simulink model "irep_force_control_m15"  (R2015a)
settings: Solver=ode3  StartTime=0.0  StopTime=inf  FixedStep=dt  RelTol=1e-3
InitFcn:
  | IREP_DEPENDENCY
  | init_omni
  | init_filters
  | init_invivo
  | init_telemanipulation
  | init_parker_xyz
  | init_magnetic_tracker
  | init_loadcell
  | init_scopes
  | init_homing
  | init_force_control
  | init_xpc_invivo_simu
undefined symbols (not defined in the file): ang_vel_scale, B_simu, beta, camera_home_voltage, counter_offset, dt, dt_trakstar, E_Y, encoder_counts, epsilon_robust_inverse, FS_LUT_TAU, FS_LUT_WE, gear_ratio, HomingFineEps, HomingRoughEps, HomingRoughVelocity, I1_primary, I1_secondary, I2_primary, I2_secondary, irep_parameters_left, irep_parameters_right, joystick_filter_coeffs, K_d, K_i, K_naive_inv, K_p, k_right, L1l, L1r, L2l, L2r, L_zeus, left_arm_home_voltage, left_x0_parallelogram, LeftArmHomingDirectionVector, LeftArmHomingIntGain, lin_vel_scale, LOADCELL_BIAS, LOADCELL_GAIN, max_conf_space_speed, N_joystick, N_pots, N_trakstar, OmegaMax, OmegaMin, orientation_epsilon, position_epsilon, pots_filter_coeffs, q_eps_backlash, quadrature_mode, r, right_arm_home_voltage, RightArmHomingDirectionVector, RightArmHomingIntGain, screw_pitch, statics_param, tau_compression_bias, tau_compression_gains, tau_neutral_deadband ... (+16)
libraries: slrtlib x39, simulink x23, xpcobsoletelib x23, xpcconteclib x23, xpcrtudplib x12, xpcmeasurementcomputinglib x6, dspswit3 x2, dspsigops x1
(part 4 of 7)

== system irep_force_control_m15/Wrench Estimation/tau sensing compensation/tau sensing compensation gain model ==
  q_bb : Inport
  tau_sensed : Inport  Port=2
  Enable : EnablePort
  friction compensation : MATLAB Function  TreatAsAtomicUnit=on
  tau_compression_bias : Constant  Value=tau_compression_bias
  tau_compression_gains : Constant  Value=tau_compression_gains
  tau_neutral_deadband : Constant  Value=tau_neutral_deadband
  tau_tension_bias : Constant  Value=tau_tension_bias
  tau_tension_gains : Constant  Value=tau_tension_gains
  tau_comp : Outport
  wires:
  tau_neutral_deadband/1 -> friction compensation/7(deadband)
  tau_compression_gains/1 -> friction compensation/4(gain_compression)
  tau_tension_gains/1 -> friction compensation/3(gain_tension)
  tau_sensed/1 -> friction compensation/2(tau_sensed)
  q_bb/1 -> friction compensation/1(q_bb)
  friction compensation/1(tau_comp) -> tau_comp/1
  tau_tension_bias/1 -> friction compensation/5(bias_tension)
  tau_compression_bias/1 -> friction compensation/6(bias_compression)

== system irep_force_control_m15/In-Vivo System/Magnetic Tracker 125 Hz/process trak1/Filter1 ==
  in : Inport
  Discrete FIR Filter : DiscreteFir  CoefSource=Input port  SampleTime=dt_trakstar  AccumDataTypeStr=Inherit: Same as product output
  Gain : Gain  Gain=1/N_trakstar  SampleTime=dt_trakstar
  trakstar_filter_coeffs : Constant  Value=trakstar_filter_coeffs  SampleTime=dt_trakstar
  out : Outport
  wires:
  Gain/1 -> out/1
  in/1 -> Discrete FIR Filter/1
  Discrete FIR Filter/1 -> Gain/1
  trakstar_filter_coeffs/1 -> Discrete FIR Filter/2

== system irep_force_control_m15/In-Vivo System/Magnetic Tracker 125 Hz/process trak2/Filter1 ==
  in : Inport
  Discrete FIR Filter : DiscreteFir  CoefSource=Input port  SampleTime=dt_trakstar  AccumDataTypeStr=Inherit: Same as product output
  Gain : Gain  Gain=1/N_trakstar  SampleTime=dt_trakstar
  trakstar_filter_coeffs : Constant  Value=trakstar_filter_coeffs  SampleTime=dt_trakstar
  out : Outport
  wires:
  trakstar_filter_coeffs/1 -> Discrete FIR Filter/2
  Discrete FIR Filter/1 -> Gain/1
  in/1 -> Discrete FIR Filter/1
  Gain/1 -> out/1

== system irep_force_control_m15/In-Vivo System/Magnetic Tracker 125 Hz/process trak3/Filter1 ==
  in : Inport
  Discrete FIR Filter : DiscreteFir  CoefSource=Input port  SampleTime=dt_trakstar  AccumDataTypeStr=Inherit: Same as product output
  Gain : Gain  Gain=1/N_trakstar  SampleTime=dt_trakstar
  trakstar_filter_coeffs : Constant  Value=trakstar_filter_coeffs  SampleTime=dt_trakstar
  out : Outport
  wires:
  Gain/1 -> out/1
  in/1 -> Discrete FIR Filter/1
  Discrete FIR Filter/1 -> Gain/1
  trakstar_filter_coeffs/1 -> Discrete FIR Filter/2

== system irep_force_control_m15/In-Vivo System/Magnetic Tracker 125 Hz/process trak4/Filter1 ==
  in : Inport
  Discrete FIR Filter : DiscreteFir  CoefSource=Input port  SampleTime=dt_trakstar  AccumDataTypeStr=Inherit: Same as product output
  Gain : Gain  Gain=1/N_trakstar  SampleTime=dt_trakstar
  trakstar_filter_coeffs : Constant  Value=trakstar_filter_coeffs  SampleTime=dt_trakstar
  out : Outport
  wires:
  trakstar_filter_coeffs/1 -> Discrete FIR Filter/2
  Discrete FIR Filter/1 -> Gain/1
  in/1 -> Discrete FIR Filter/1
  Gain/1 -> out/1

== system irep_force_control_m15/Trajectory Planner/Left Arm/High Level/Actuation Compensation ==
  q des : Inport
  conf space : Inport  Port=2
  Enable : EnablePort
  1/stiffness : Gain  Gain=K_naive_inv  Multiplication=Matrix(K*u)  SampleTime=dt
  Compute Taus : Subsystem
  Grad U1 : Subsystem
  Grad U2 : Subsystem
  Mux : Mux  Inputs=2
  Mux1 : Mux  Inputs=3
  Parallelogram Backlash Compensatior : Subsystem  TreatAsAtomicUnit=on
  comp perc : Gain  Gain=diag([0.8 0.8 0.8 0.8])  Multiplication=Matrix(K*u)  SampleTime=dt
  padding 2 for wrist and gripper : Constant  Value=zeros(2,1)  SampleTime=dt
  epsilon : Outport
  wires:
  conf space/1 -> Grad U1/1(conf space), Compute Taus/2(In2), Grad U2/1(conf space)
  q des/1 -> Grad U2/2(q), Grad U1/2(q), Parallelogram Backlash Compensatior/1(q des)
  Grad U1/1(grad_U) -> Mux/1
  Grad U2/1(grad_U) -> Mux/2
  Mux/1 -> Compute Taus/1(In1)
  Compute Taus/1(tau) -> 1/stiffness/1
  Parallelogram Backlash Compensatior/1(epsilon) -> Mux1/1
  1/stiffness/1 -> comp perc/1  "epsilon"
  padding 2 for wrist and gripper/1 -> Mux1/3
  comp perc/1 -> Mux1/2
  Mux1/1 -> epsilon/1

== system irep_force_control_m15/Trajectory Planner/Left Arm/High Level/Configuration Space ==
  Enable : EnablePort
  Enable Parallelogram : Constant  Value=0  SampleTime=dt
  Enable Stem : Constant  Value=0  SampleTime=dt
  Mux : Mux  Inputs=3
  Parallelogram : Subsystem  TreatAsAtomicUnit=on
  Stem : Subsystem  TreatAsAtomicUnit=on
  b0 : Constant  Value=0  SampleTime=dt
  "b1 dot, psi dot" : Outport  InitialOutput=zeros(8,1)
  wires:
  Enable Stem/1 -> Stem/Enable
  Enable Parallelogram/1 -> Parallelogram/Enable
  Mux/1 -> "b1 dot, psi dot"/1
  b0/1 -> Mux/1
  Parallelogram/1(b1) -> Mux/2
  Stem/1(psi dot) -> Mux/3

== system irep_force_control_m15/Trajectory Planner/Left Arm/High Level/Inverse Istantaneous Kinematics ==
  In1 : Inport
  sensors : Inport  Port=2
  Master : Inport  Port=3
  5-Bar Inverse Kinematics : MATLAB Function  TreatAsAtomicUnit=on
  Bus Creator : BusCreator  Inputs=3
  Bus Creator1 : BusCreator
  Bus Selector : BusSelector  OutputSignals=q.Parker insertion stage
  Coordination Module : Subsystem
  Demux : Demux  Outputs=[1 2 5]
  Enable Gripper : Constant  Value=0  SampleTime=dt
  Integrator 3 : DiscreteIntegrator  InitialCondition=[left_x0_parallelogram z0_parallelogram]  SampleTime=dt  LimitOutput=on  UpperSaturationLimit=[-x0_parallelogram z0_parallelogram_max]  LowerSaturationLimit=[-x0_parallelogram_max z0_parallelogram]
  Integrator 4 : DiscreteIntegrator  InitialCondition=[pi/2;0;pi/2;0;0]  SampleTime=dt  LimitOutput=on  UpperSaturationLimit=[theta_max inf theta_max inf wrist_max]  LowerSaturationLimit=[theta_min1 -inf theta_min2 -inf wrist_min]
  Jaw Open/Close Module : Subsystem  TreatAsAtomicUnit=on
  Saturation : Saturate  UpperLimit=20  LowerLimit=0
  Snake inverse kinematics : MATLAB Function  TreatAsAtomicUnit=on
  q des : Outport
  conf space : Outport  Port=2
  b0 dot left : Outport  Port=3
  wires:
  Integrator 4/1 -> Snake inverse kinematics/1(psi), Bus Creator/3  "psi curr"
  Bus Creator/1 -> conf space/1
  In1/1 -> Demux/1
  Bus Creator1/1 -> q des/1
  Jaw Open/Close Module/1(q9) -> Bus Creator1/4  "q9"
  Coordination Module/2("q2, q3") -> Bus Creator1/2  "q2, q3"
  Coordination Module/1(q1) -> Saturation/1  "q1"
  Integrator 3/1 -> 5-Bar Inverse Kinematics/1(b1), Coordination Module/1(b1), Bus Creator/2  "b1 curr"
  5-Bar Inverse Kinematics/1(q) -> Coordination Module/2(q par)
  sensors/1 -> Bus Selector/1
  Enable Gripper/1 -> Jaw Open/Close Module/Enable
  Saturation/1 -> Bus Creator1/1
  Snake inverse kinematics/1(q) -> Bus Creator1/3
  Bus Selector/1 -> Bus Creator/1  "<Parker insertion stage>"
  Demux/3 -> Integrator 4/1
  Demux/2 -> Integrator 3/1  "psi dot"
  Demux/1 -> b0 dot left/1  "b1 dot"
  Master/1 -> Jaw Open/Close Module/1(sensors)

== system irep_force_control_m15/Trajectory Planner/Left Arm/High Level/Task Space ==
  note: IREP Task Space Module v 0.2 - © 2011 Andrea Bajo, Nabil Simaan
  Master : Inport
  "b1 curr, psi curr" : Inport  Port=2
  sensors : Inport  Port=3
  Enable : EnablePort
  Bus Creator : BusCreator  Inputs=2
  Bus Selector : BusSelector  OutputSignals=p in world,R in world
  Compute Weigths : Subsystem  TreatAsAtomicUnit=on
  Desired Twist Module : Subsystem
  Direct Kinematics IREP : Subsystem  TreatAsAtomicUnit=on
  Jxpsi Inverse IREP : Subsystem  TreatAsAtomicUnit=on
  Receive Desired Pose from MTM : Subsystem
  pose cur quat : MATLAB Function  TreatAsAtomicUnit=on
  right task space scope : Subsystem
  "b1 dot, psi dot" : Outport  PortDimensions=8  InitialOutput=zeros(8,1)
  current_pose : Outport  Port=2  PortDimensions=7  InitialOutput=[zeros(3,1);1;0;0;0]
  wires:
  "b1 curr, psi curr"/1 -> Direct Kinematics IREP/1("b1, psi"), Jxpsi Inverse IREP/3("b1, psi"), Compute Weigths/2(conf space)
  Receive Desired Pose from MTM/1("pose, flags") -> Desired Twist Module/2(des pose), [L_pose_des]
  Direct Kinematics IREP/1(Current Pose) -> Desired Twist Module/1(current pose), Bus Selector/1
  Master/1 -> Receive Desired Pose from MTM/1(Master)
  Jxpsi Inverse IREP/1(conf dot des) -> "b1 dot, psi dot"/1
  Desired Twist Module/1(x des) -> Jxpsi Inverse IREP/1(x des)
  Compute Weigths/1(weights) -> Jxpsi Inverse IREP/2(weights)
  [L_pose_des] -> right task space scope/1(In)
  sensors/1 -> Compute Weigths/1(sensors)
  Bus Selector/1 -> Bus Creator/1  "<p in world>"
  Bus Selector/2 -> pose cur quat/1(R)  "<R in world>"
  pose cur quat/1(quat) -> Bus Creator/2
  Bus Creator/1 -> current_pose/1

== system irep_force_control_m15/Trajectory Planner/Left Arm/Low Level/Home Procedure ==
  sensors : Inport
  Enable : EnablePort
  Bus Selector : BusSelector  OutputSignals=A/D signals.left arm pots
  Demux : Demux  Outputs=[9 1]
  Fine Homing - Integral Control : Subsystem
  Fine_Rough_Homing_Switch : MATLAB Function  TreatAsAtomicUnit=on
  Homing Direction : Gain  Gain=diag(LeftArmHomingDirectionVector)  Multiplication=Matrix(K*u)  SampleTime=dt
  Homing Flags : Subsystem
  HomingRoughEps : Constant  Value=HomingRoughEps  SampleTime=dt
  HomingRoughVelocity : Constant  Value=HomingRoughVelocity  SampleTime=dt
  Select Homing Joint : Gain  Gain=diag([1;1;1;1;1;1;1;1;1])  Multiplication=Matrix(K*u)  SampleTime=dt
  Sum : Sum  Inputs=|+-  SampleTime=dt
  Sum1 : Sum  Inputs=|++
  Terminator : Terminator
  Unit Delay : UnitDelay  InitialCondition=zeros(9,1)  SampleTime=-1
  Unit Delay1 : UnitDelay  InitialCondition=false(9,1)  SampleTime=-1
  dt : Constant  Value=dt  SampleTime=dt
  home voltage : Constant  Value=left_arm_home_voltage  SampleTime=dt
  q des : Outport  InitialOutput=zeros(9,1)
  wires:
  sensors/1 -> Bus Selector/1
  Sum/1 -> Select Homing Joint/1
  home voltage/1 -> Sum/1
  Bus Selector/1 -> Demux/1  "<left arm pots>"
  Demux/1 -> Sum/2
  Demux/2 -> Terminator/1
  Select Homing Joint/1 -> Homing Direction/1
  HomingRoughVelocity/1 -> Fine_Rough_Homing_Switch/4(HomingVel)
  Unit Delay1/1 -> Fine_Rough_Homing_Switch/6(PrevHomedJoint)
  Fine_Rough_Homing_Switch/3(HomedJoint) -> Unit Delay1/1
  HomingRoughEps/1 -> Fine_Rough_Homing_Switch/3(ERROR_eps)
  dt/1 -> Fine_Rough_Homing_Switch/2(dt)
  Unit Delay/1 -> Fine_Rough_Homing_Switch/5(q_cur)
  Fine_Rough_Homing_Switch/2(q_des) -> Unit Delay/1, Sum1/2
  Fine_Rough_Homing_Switch/1(EnableFineHoming) -> Fine Homing - Integral Control/Enable
  Fine Homing - Integral Control/1(q_des_fine) -> Sum1/1
  Sum1/1 -> q des/1
  Homing Direction/1 -> Fine_Rough_Homing_Switch/1(error), Fine Homing - Integral Control/1(error), Homing Flags/1(u)

== system irep_force_control_m15/Trajectory Planner/Left Arm/Low Level/Joint Space ==
  Enable : EnablePort
  q desired : Constant  Value=zeros(9,1)  SampleTime=dt
  q des : Outport
  wires:
  q desired/1 -> q des/1

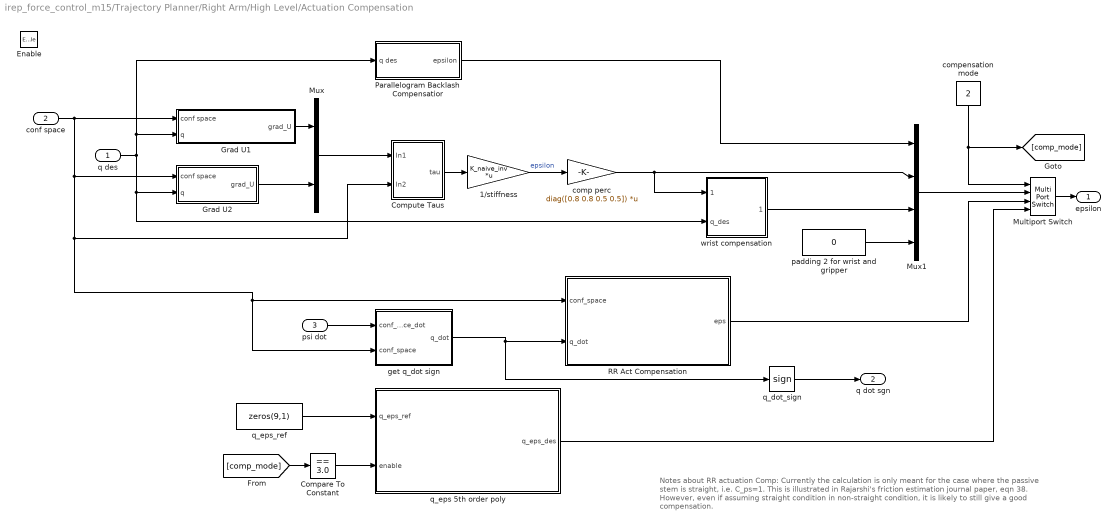
== system irep_force_control_m15/Trajectory Planner/Right Arm/High Level/Actuation Compensation ==
  note: Notes about RR actuation Comp:
      | Currently the calculation is only meant for the case where the passive stem is straight, i.e. C_ps=1.
      | This is illustrated in Rajarshi's friction estimation journal paper, eqn 38.
      | However, even if assuming straight condition in non-straight condition,
      | it is likely to still give a good compensation.
  q des : Inport
  conf space : Inport  Port=2
  psi dot : Inport  Port=3
  Enable : EnablePort
  1/stiffness : Gain  Gain=K_naive_inv  Multiplication=Matrix(K*u)  SampleTime=dt
  Compare To Constant : simulink/Logic and Bit Operations/Compare To Constant  relop===  const=3.0  OutDataTypeStr=uint8
  Compute Taus : Subsystem
  Grad U1 : Subsystem
  Grad U2 : Subsystem
  Multiport Switch : MultiPortSwitch
  Mux : Mux  Inputs=2
  Mux1 : Mux
  Parallelogram Backlash Compensatior : Subsystem  TreatAsAtomicUnit=on
  RR Act Compensation : MATLAB Function  TreatAsAtomicUnit=on
  comp perc : Gain  Gain=diag([0.8 0.8 0.5 0.5])  Multiplication=Matrix(K*u)  SampleTime=dt
  compensation mode : Constant  Value=2
  get q_dot sign : Subsystem
  padding 2 for wrist and gripper : Constant  Value=0  SampleTime=dt
  q_dot_sign : Signum
  q_eps 5th order poly : Subsystem
  q_eps_ref : Constant  Value=zeros(9,1)  SampleTime=dt
  wrist compensation : MATLAB Function  TreatAsAtomicUnit=on
  epsilon : Outport
  q dot sgn : Outport  Port=2
  wires:
  conf space/1 -> Grad U1/1(conf space), Grad U2/1(conf space), Compute Taus/2(In2), RR Act Compensation/1(conf_space), get q_dot sign/2(conf_space)
  q des/1 -> Grad U1/2(q), Parallelogram Backlash Compensatior/1(q des), Grad U2/2(q), wrist compensation/2(q_des)
  Grad U1/1(grad_U) -> Mux/1
  Grad U2/1(grad_U) -> Mux/2
  Mux/1 -> Compute Taus/1(In1)
  Compute Taus/1(tau) -> 1/stiffness/1
  Parallelogram Backlash Compensatior/1(epsilon) -> Mux1/1
  1/stiffness/1 -> comp perc/1  "epsilon"
  comp perc/1 -> Mux1/2, wrist compensation/1(epsilon)
  padding 2 for wrist and gripper/1 -> Mux1/4
  wrist compensation/1(q_wrist) -> Mux1/3
  Multiport Switch/1 -> epsilon/1
  Mux1/1 -> Multiport Switch/2
  compensation mode/1 -> Multiport Switch/1, [comp_mode]
  RR Act Compensation/1(eps) -> Multiport Switch/3
  q_eps_ref/1 -> q_eps 5th order poly/1(q_eps_ref)
  Compare To Constant/1 -> q_eps 5th order poly/2(enable)
  q_eps 5th order poly/1(q_eps_des) -> Multiport Switch/4
  [comp_mode] -> Compare To Constant/1
  psi dot/1 -> get q_dot sign/1(conf_space_dot)
  get q_dot sign/1(q_dot) -> q_dot_sign/1, RR Act Compensation/2(q_dot)
  q_dot_sign/1 -> q dot sgn/1

== system irep_force_control_m15/Trajectory Planner/Right Arm/High Level/Configuration Space ==
  Enable : EnablePort
  Enable Parallelogram : Constant  Value=0  SampleTime=dt
  Enable Stem : Constant  Value=0  SampleTime=dt
  Mux : Mux  Inputs=3
  Parallelogram : Subsystem  TreatAsAtomicUnit=on
  Stem : Subsystem  TreatAsAtomicUnit=on
  XYZ : Constant  Value=0  SampleTime=dt
  "b1 dot, psi dot" : Outport  PortDimensions=8  InitialOutput=zeros(8,1)
  wires:
  Mux/1 -> "b1 dot, psi dot"/1
  Enable Parallelogram/1 -> Parallelogram/Enable
  Enable Stem/1 -> Stem/Enable
  Stem/1(psi dot) -> Mux/3
  Parallelogram/1(b1) -> Mux/2
  XYZ/1 -> Mux/1

== system irep_force_control_m15/Trajectory Planner/Right Arm/High Level/Inverse Istantaneous Kinematics ==
  PSI dot : Inport
  sensors : Inport  Port=2
  Master : Inport  Port=3
  5-Bar Inverse Kinematics : MATLAB Function  TreatAsAtomicUnit=on
  Bus Creator : BusCreator  Inputs=3
  Bus Selector : BusSelector  OutputSignals=q.Parker insertion stage
  Coordination Module : Subsystem
  Demux : Demux  Outputs=[1 2 5]
  Enable Gripper : Constant  Value=0  SampleTime=dt
  Integrator 3 : DiscreteIntegrator  InitialCondition=[x0_parallelogram z0_parallelogram]  SampleTime=dt  LimitOutput=on  UpperSaturationLimit=[x0_parallelogram_max z0_parallelogram_max]  LowerSaturationLimit=[x0_parallelogram z0_parallelogram]
  Integrator 4 : DiscreteIntegrator  InitialCondition=[pi/2;0;pi/2;0;0]  SampleTime=dt  LimitOutput=on  UpperSaturationLimit=[theta_max inf theta_max inf wrist_max]  LowerSaturationLimit=[theta_min1 -inf theta_min2 -inf wrist_min]
  Jaw Open/Close Module : Subsystem  TreatAsAtomicUnit=on
  Mux : Mux
  Saturation : Saturate  UpperLimit=30  LowerLimit=0
  Snake inverse position : MATLAB Function  TreatAsAtomicUnit=on
  q des : Outport
  conf space : Outport  Port=2  PortDimensions=8
  b0_dot_right : Outport  Port=3
  wires:
  5-Bar Inverse Kinematics/1(q) -> Coordination Module/2(q par)
  Integrator 3/1 -> [b1], 5-Bar Inverse Kinematics/1(b1), Coordination Module/1(b1)  "b1 curr"
  Coordination Module/1(q1) -> Saturation/1  "q1"
  Jaw Open/Close Module/1(q9) -> Mux/4  "q9"
  Mux/1 -> q des/1
  PSI dot/1 -> Demux/1
  Bus Creator/1 -> conf space/1
  Integrator 4/1 -> Bus Creator/3, Snake inverse position/1(psi)  "psi curr"
  Coordination Module/2("q2, q3") -> Mux/2  "q2, q3"
  sensors/1 -> Bus Selector/1
  Enable Gripper/1 -> Jaw Open/Close Module/Enable
  [b1] -> Bus Creator/2
  Bus Selector/1 -> Bus Creator/1  "<Parker insertion stage>"
  Demux/3 -> Integrator 4/1  "psi dot"
  Demux/2 -> Integrator 3/1  "b1 dot"
  Demux/1 -> b0_dot_right/1  "b0 dot"
  Saturation/1 -> Mux/1
  Snake inverse position/1(q) -> Mux/3
  Master/1 -> Jaw Open/Close Module/1(sensors)

== system irep_force_control_m15/Trajectory Planner/Right Arm/High Level/Task Space ==
  note: IREP Task Space Module v 0.2 - © 2011 Andrea Bajo, Nabil Simaan
  Master : Inport
  "b1 curr, psi curr" : Inport  Port=2
  sensors : Inport  Port=3
  Enable : EnablePort
  Bus Creator : BusCreator  Inputs=2
  Bus Selector : BusSelector  OutputSignals=p in world,R in world
  Compute Weigths : Subsystem  TreatAsAtomicUnit=on
  Desired Twist Module : Subsystem
  Direct Kinematics IREP : Subsystem  TreatAsAtomicUnit=on
  Jxpsi Inverse IREP : Subsystem  TreatAsAtomicUnit=on
  Receive Desired Pose from MTM : Subsystem
  pose cur quat : MATLAB Function  TreatAsAtomicUnit=on
  right task space scope : Subsystem
  "b0 dot, b1 dot, psi dot" : Outport  PortDimensions=8  InitialOutput=zeros(8,1)
  current_pose : Outport  Port=2  PortDimensions=7  InitialOutput=[zeros(3,1);1;0;0;0]
  wires:
  "b1 curr, psi curr"/1 -> Direct Kinematics IREP/1("b1, psi"), Compute Weigths/2(conf space), Jxpsi Inverse IREP/3("b1, psi")
  Receive Desired Pose from MTM/1("pose, flags") -> Desired Twist Module/2(des pose), [R_Pose_des]
  Direct Kinematics IREP/1(Current Pose) -> Desired Twist Module/1(current pose), Bus Selector/1
  Master/1 -> Receive Desired Pose from MTM/1(Master)
  Jxpsi Inverse IREP/1(conf dot des) -> "b0 dot, b1 dot, psi dot"/1
  Desired Twist Module/1(x des) -> Jxpsi Inverse IREP/1(x des)
  Compute Weigths/1(weights) -> Jxpsi Inverse IREP/2(weights)
  [R_Pose_des] -> right task space scope/1(des)
  sensors/1 -> Compute Weigths/1(sensors)
  Bus Creator/1 -> current_pose/1
  Bus Selector/1 -> Bus Creator/1  "<p in world>"
  Bus Selector/2 -> pose cur quat/1(R)  "<R in world>"
  pose cur quat/1(quat) -> Bus Creator/2

== system irep_force_control_m15/Trajectory Planner/Right Arm/High Level/delay ==
  In1 : Inport
  Bus Creator : BusCreator
  Demux : Demux  Outputs=[1,2,5,1]
  Unit Delay : UnitDelay  InitialCondition=zeros(9,1)  SampleTime=-1
  Out1 : Outport
  wires:
  Unit Delay/1 -> Demux/1
  In1/1 -> Unit Delay/1
  Bus Creator/1 -> Out1/1
  Demux/1 -> Bus Creator/1  "q1"
  Demux/2 -> Bus Creator/2  "q2;q3"
  Demux/3 -> Bus Creator/3  "q_snake"
  Demux/4 -> Bus Creator/4  "q9"

== system irep_force_control_m15/Trajectory Planner/Right Arm/Low Level/Home Procedure ==
  sensors : Inport
  Enable : EnablePort
  Bus Selector : BusSelector  OutputSignals=A/D signals.right arm pots
  Demux : Demux  Outputs=[9 1]
  Fine Homing - Integral Control : Subsystem
  Fine_Rough_Homing_Switch : MATLAB Function  TreatAsAtomicUnit=on
  Homing Completion : MATLAB Function  TreatAsAtomicUnit=on
  Homing Direction : Gain  Gain=diag(RightArmHomingDirectionVector)  Multiplication=Matrix(K*u)  SampleTime=dt
  HomingFineEps : Constant  Value=HomingFineEps  SampleTime=dt
  HomingRoughEps : Constant  Value=HomingRoughEps  SampleTime=dt
  HomingRoughVelocity : Constant  Value=HomingRoughVelocity  SampleTime=dt
  Select Homing Joint : Gain  Gain=diag([1;1;1;1;1;1;1;0;0])  Multiplication=Matrix(K*u)  SampleTime=dt
  Sum : Sum  Inputs=|+-  SampleTime=dt
  Sum1 : Sum  Inputs=|++
  Terminator : Terminator
  Terminator1 : Terminator
  Unit Delay : UnitDelay  InitialCondition=zeros(9,1)  SampleTime=-1
  Unit Delay1 : UnitDelay  InitialCondition=false(9,1)  SampleTime=-1
  dt : Constant  Value=dt  SampleTime=dt
  home voltage : Constant  Value=right_arm_home_voltage  SampleTime=dt
  q des : Outport  InitialOutput=zeros(9,1)
  wires:
  sensors/1 -> Bus Selector/1
  Sum/1 -> Select Homing Joint/1
  home voltage/1 -> Sum/1
  Bus Selector/1 -> Demux/1  "<right arm pots>"
  Demux/1 -> Sum/2
  Demux/2 -> Terminator/1
  Homing Completion/1(Homed) -> Terminator1/1
  Select Homing Joint/1 -> Homing Direction/1
  HomingRoughVelocity/1 -> Fine_Rough_Homing_Switch/4(HomingVel)
  Unit Delay1/1 -> Fine_Rough_Homing_Switch/6(PrevHomedJoint)
  Fine_Rough_Homing_Switch/3(HomedJoint) -> Unit Delay1/1
  HomingRoughEps/1 -> Fine_Rough_Homing_Switch/3(ERROR_eps)
  dt/1 -> Fine_Rough_Homing_Switch/2(dt)
  Unit Delay/1 -> Fine_Rough_Homing_Switch/5(q_cur)
  Fine_Rough_Homing_Switch/2(q_des) -> Unit Delay/1, Sum1/2
  Fine_Rough_Homing_Switch/1(EnableFineHoming) -> Fine Homing - Integral Control/Enable
  Fine Homing - Integral Control/1(q_des_fine) -> Sum1/1
  Sum1/1 -> q des/1
  Homing Direction/1 -> Homing Completion/1(u), Fine_Rough_Homing_Switch/1(error), Fine Homing - Integral Control/1(error)
  HomingFineEps/1 -> Homing Completion/2(EPS)

== system irep_force_control_m15/Trajectory Planner/Right Arm/Low Level/Joint Space ==
  Enable : EnablePort
  q desired : Constant  Value=zeros(9,1)  SampleTime=dt
  q des : Outport
  wires:
  q desired/1 -> q des/1

== system irep_force_control_m15/Trajectory Planner/UDP_SendTo_MTM/Left_UDP/pose convert ==
  pose_q : Inport
  Bus Creator : BusCreator  Inputs=2
  Bus Selector4 : BusSelector  OutputSignals=p in world,quat
  Quaternion To Rotation : MATLAB Function  TreatAsAtomicUnit=on
  pose_R : Outport
  wires:
  Bus Creator/1 -> pose_R/1
  Bus Selector4/1 -> Bus Creator/1  "<p in world>"
  Quaternion To Rotation/1(R) -> Bus Creator/2  "R in world"
  pose_q/1 -> Bus Selector4/1
  Bus Selector4/2 -> Quaternion To Rotation/1(quat)  "<quat>"

== system irep_force_control_m15/Trajectory Planner/UDP_SendTo_MTM/Left_UDP/pose_curr_scope ==
  left : Inport
  q9 : Inport  Port=2
  Bus Selector1 : BusSelector  OutputSignals=p in world,R in world
  Gain2 : Gain
  Mux1 : Mux
  R_to_axis_angle1 : MATLAB Function  TreatAsAtomicUnit=on
  left  task cur : slrtlib/Displays and Logging/Scope   scopeno=11  scopetype=Host  autostart=on  viewmode=Numerical  formatstr=scope_format_left_task_space_cur  grid=on  ylimits=[0,0]  nosamples=10  noprepostsamples=0  interleave=1  triggermode=FreeRun  triggersignal=1  trigsignalfromport=off  triggerlevel=0.0  triggerslope=Either  triggerscope=1  triggersample=0  filename=weights1.dat  mode=Lazy  writesize=512  autorestart=off  dynamicfilemode=off  maxwritefilesize=512*1024^2
  wires:
  Mux1/1 -> Gain2/1
  left/1 -> Bus Selector1/1
  Bus Selector1/2 -> R_to_axis_angle1/1(R)  "<R in world>"
  Gain2/1 -> left  task cur/1
  Bus Selector1/1 -> Mux1/1  "<p in world>"
  R_to_axis_angle1/1(n_vec) -> Mux1/2
  R_to_axis_angle1/2(theta) -> Mux1/3
  q9/1 -> Mux1/4

== system irep_force_control_m15/Trajectory Planner/UDP_SendTo_MTM/Left_UDP/select q9 ==
  qdes : Inport
  Demux1 : Demux  Outputs=9
  Terminator{,1..7} (8 alike) : Terminator
  q9 : Outport
  wires:
  Demux1/9 -> q9/1
  qdes/1 -> Demux1/1
  Demux1/8 -> Terminator7/1
  Demux1/7 -> Terminator6/1
  Demux1/6 -> Terminator5/1
  Demux1/5 -> Terminator4/1
  Demux1/4 -> Terminator3/1
  Demux1/3 -> Terminator2/1
  Demux1/2 -> Terminator1/1
  Demux1/1 -> Terminator/1

== system irep_force_control_m15/Trajectory Planner/UDP_SendTo_MTM/Right_UDP/pose convert ==
  pose_q : Inport
  Bus Creator : BusCreator  Inputs=2
  Bus Selector4 : BusSelector  OutputSignals=p in world,quat
  Quaternion To Rotation : MATLAB Function  TreatAsAtomicUnit=on
  pose_R : Outport
  wires:
  Bus Selector4/2 -> Quaternion To Rotation/1(quat)  "<quat>"
  pose_q/1 -> Bus Selector4/1
  Quaternion To Rotation/1(R) -> Bus Creator/2  "R in world"
  Bus Selector4/1 -> Bus Creator/1  "<p in world>"
  Bus Creator/1 -> pose_R/1

== system irep_force_control_m15/Trajectory Planner/UDP_SendTo_MTM/Right_UDP/pose_curr_scope ==
  right : Inport
  q9 : Inport  Port=2
  Bus Selector5 : BusSelector  OutputSignals=p in world,R in world
  Gain1 : Gain
  Mux2 : Mux
  R_to_axis_angle2 : MATLAB Function  TreatAsAtomicUnit=on
  right task cur : slrtlib/Displays and Logging/Scope   scopeno=27  scopetype=Host  autostart=on  viewmode=Numerical  formatstr=scope_format_right_task_space_cur  grid=on  ylimits=[0,0]  nosamples=10  noprepostsamples=0  interleave=1  triggermode=FreeRun  triggersignal=1  trigsignalfromport=off  triggerlevel=0.0  triggerslope=Either  triggerscope=1  triggersample=0  filename=weights1.dat  mode=Lazy  writesize=512  autorestart=off  dynamicfilemode=off  maxwritefilesize=512*1024^2
  wires:
  Mux2/1 -> Gain1/1
  right/1 -> Bus Selector5/1
  Bus Selector5/2 -> R_to_axis_angle2/1(R)  "<R in world>"
  Gain1/1 -> right task cur/1
  Bus Selector5/1 -> Mux2/1  "<p in world>"
  R_to_axis_angle2/1(n_vec) -> Mux2/2
  R_to_axis_angle2/2(theta) -> Mux2/3
  q9/1 -> Mux2/4

== system irep_force_control_m15/Trajectory Planner/UDP_SendTo_MTM/Right_UDP/select q9 ==
  qdes : Inport
  Demux1 : Demux  Outputs=9
  Terminator{,1..7} (8 alike) : Terminator
  q9 : Outport
  wires:
  Demux1/1 -> Terminator/1
  Demux1/2 -> Terminator1/1
  Demux1/3 -> Terminator2/1
  Demux1/4 -> Terminator3/1
  Demux1/5 -> Terminator4/1
  Demux1/6 -> Terminator5/1
  Demux1/7 -> Terminator6/1
  Demux1/8 -> Terminator7/1
  qdes/1 -> Demux1/1
  Demux1/9 -> q9/1

== system irep_force_control_m15/Trajectory Planner/UDP_SendTo_MTM/Right_UDP/to file ==
  right : Inport
  Enable : EnablePort
  Joint Space Info File : slrtlib/Displays and Logging/Scope   scopeno=28  scopetype=File  autostart=on  viewmode=Numerical  formatstr="'tau: %8.3f,     %8.3f,     %8.3f,     %8.3f,     %8.3f,     %8.3f'"  grid=on  ylimits=[0,0]  nosamples=100000  noprepostsamples=0  interleave=1  triggermode=FreeRun  triggersignal=1  trigsignalfromport=off  triggerlevel=0.0  triggerslope=Either  triggerscope=1  triggersample=0  filename=IREPR.dat  mode=Lazy  writesize=512  autorestart=off  dynamicfilemode=off  maxwritefilesize=512*1024^2
  wires:
  right/1 -> Joint Space Info File/1

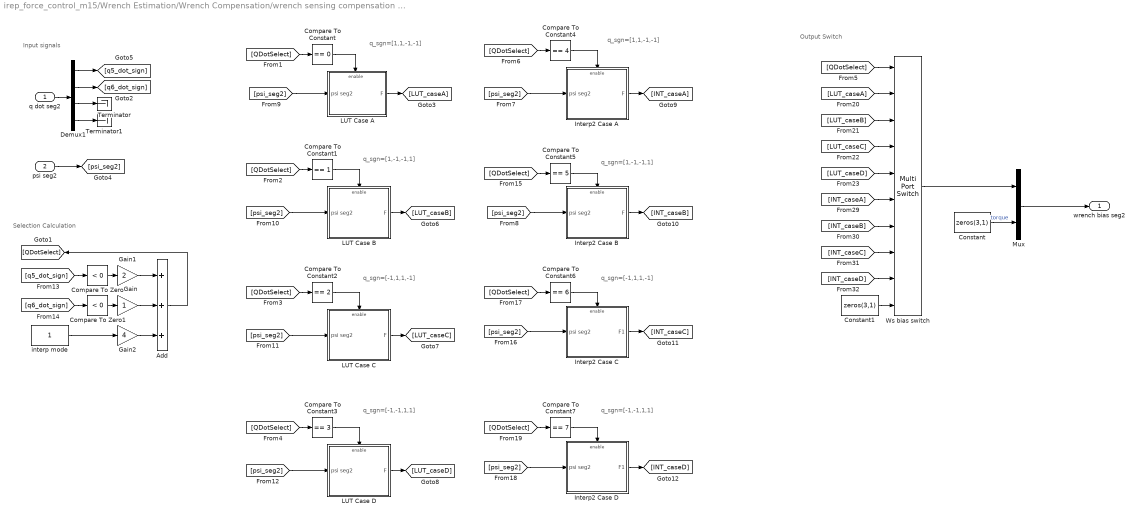
== system irep_force_control_m15/Wrench Estimation/Wrench Compensation/wrench sensing compensation LUT/wrench seg2 bias LUT ==
  note: q_sgn=[1,1,-1,-1]
  note: Output Switch
  note: Selection Calculation
  note: Input signals
  note: q_sgn=[1,-1,-1,1]
  note: q_sgn=[-1,1,1,-1]
  note: q_sgn=[-1,-1,1,1]
  note: q_sgn=[1,1,-1,-1]
  note: q_sgn=[1,-1,-1,1]
  note: q_sgn=[-1,1,1,-1]
  note: q_sgn=[-1,-1,1,1]
  q dot seg2 : Inport
  psi seg2 : Inport  Port=2
  Add : Sum  Inputs=+++
  Compare To Constant : simulink/Logic and Bit Operations/Compare To Constant  relop===  const=0  OutDataTypeStr=boolean
  Compare To Constant1 : simulink/Logic and Bit Operations/Compare To Constant  relop===  const=1  OutDataTypeStr=boolean
  Compare To Constant2 : simulink/Logic and Bit Operations/Compare To Constant  relop===  const=2  OutDataTypeStr=boolean
  Compare To Constant3 : simulink/Logic and Bit Operations/Compare To Constant  relop===  const=3  OutDataTypeStr=boolean
  Compare To Constant4 : simulink/Logic and Bit Operations/Compare To Constant  relop===  const=4  OutDataTypeStr=boolean
  Compare To Constant5 : simulink/Logic and Bit Operations/Compare To Constant  relop===  const=5  OutDataTypeStr=boolean
  Compare To Constant6 : simulink/Logic and Bit Operations/Compare To Constant  relop===  const=6  OutDataTypeStr=boolean
  Compare To Constant7 : simulink/Logic and Bit Operations/Compare To Constant  relop===  const=7  OutDataTypeStr=boolean
  Compare To Zero : simulink/Logic and Bit Operations/Compare To Zero  relop=<  OutDataTypeStr=uint8
  Compare To Zero1 : simulink/Logic and Bit Operations/Compare To Zero  relop=<  OutDataTypeStr=uint8
  Constant : Constant  Value=zeros(3,1)
  Constant1 : Constant  Value=zeros(3,1)
  Demux1 : Demux
  Gain : Gain
  Gain1 : Gain  Gain=2
  Gain2 : Gain  Gain=4
  Interp2 Case A : Subsystem
  Interp2 Case B : Subsystem
  Interp2 Case C : Subsystem
  Interp2 Case D : Subsystem
  LUT Case A : Subsystem
  LUT Case B : Subsystem
  LUT Case C : Subsystem
  LUT Case D : Subsystem
  Mux : Mux  Inputs=2
  Terminator : Terminator
  Terminator1 : Terminator
  Ws bias switch : MultiPortSwitch  DataPortOrder=Specify indices  DataPortIndices={0,1,2,3,4,5,6,7,8}
  interp mode : Constant
  wrench bias seg2 : Outport
  wires:
  Mux/1 -> wrench bias seg2/1
  psi seg2/1 -> [psi_seg2]
  q dot seg2/1 -> Demux1/1
  Demux1/1 -> [q5_dot_sign]
  Demux1/2 -> [q6_dot_sign]
  Demux1/3 -> Terminator/1
  Demux1/4 -> Terminator1/1
  Constant/1 -> Mux/2  "torque"
  Compare To Constant/1 -> LUT Case A/Enable
  Ws bias switch/1 -> Mux/1
  [psi_seg2] -> LUT Case A/1(psi seg2)
  [psi_seg2] -> LUT Case B/1(psi seg2)
  [psi_seg2] -> LUT Case C/1(psi seg2)
  [psi_seg2] -> LUT Case D/1(psi seg2)
  [q5_dot_sign] -> Compare To Zero/1
  [q6_dot_sign] -> Compare To Zero1/1
  Compare To Zero/1 -> Gain1/1
  Compare To Zero1/1 -> Gain/1
  Gain1/1 -> Add/1
  Gain/1 -> Add/2
  Add/1 -> [QDotSelect]
  [QDotSelect] -> Compare To Constant/1
  Compare To Constant1/1 -> LUT Case B/Enable
  [QDotSelect] -> Compare To Constant1/1
  Compare To Constant2/1 -> LUT Case C/Enable
  [QDotSelect] -> Compare To Constant2/1
  Compare To Constant3/1 -> LUT Case D/Enable
  [QDotSelect] -> Compare To Constant3/1
  [QDotSelect] -> Ws bias switch/1
  Compare To Constant4/1 -> Interp2 Case A/Enable
  [psi_seg2] -> Interp2 Case A/1(psi seg2)
  [QDotSelect] -> Compare To Constant4/1
  [psi_seg2] -> Interp2 Case B/1(psi seg2)
  Compare To Constant5/1 -> Interp2 Case B/Enable
  [QDotSelect] -> Compare To Constant5/1
  [psi_seg2] -> Interp2 Case C/1(psi seg2)
  Compare To Constant6/1 -> Interp2 Case C/Enable
  [QDotSelect] -> Compare To Constant6/1
  [psi_seg2] -> Interp2 Case D/1(psi seg2)
  Compare To Constant7/1 -> Interp2 Case D/Enable
  [QDotSelect] -> Compare To Constant7/1
  LUT Case A/1(F) -> [LUT_caseA]
  LUT Case B/1(F) -> [LUT_caseB]
  LUT Case C/1(F) -> [LUT_caseC]
  LUT Case D/1(F) -> [LUT_caseD]
  Interp2 Case A/1(F) -> [INT_caseA]
  Interp2 Case B/1(F) -> [INT_caseB]
  Interp2 Case C/1(F1) -> [INT_caseC]
  Interp2 Case D/1(F1) -> [INT_caseD]
  [LUT_caseA] -> Ws bias switch/2
  [LUT_caseB] -> Ws bias switch/3
  [LUT_caseC] -> Ws bias switch/4
  [LUT_caseD] -> Ws bias switch/5
  Gain2/1 -> Add/3
  interp mode/1 -> Gain2/1
  Constant1/1 -> Ws bias switch/10
  [INT_caseA] -> Ws bias switch/6
  [INT_caseC] -> Ws bias switch/8
  [INT_caseB] -> Ws bias switch/7
  [INT_caseD] -> Ws bias switch/9

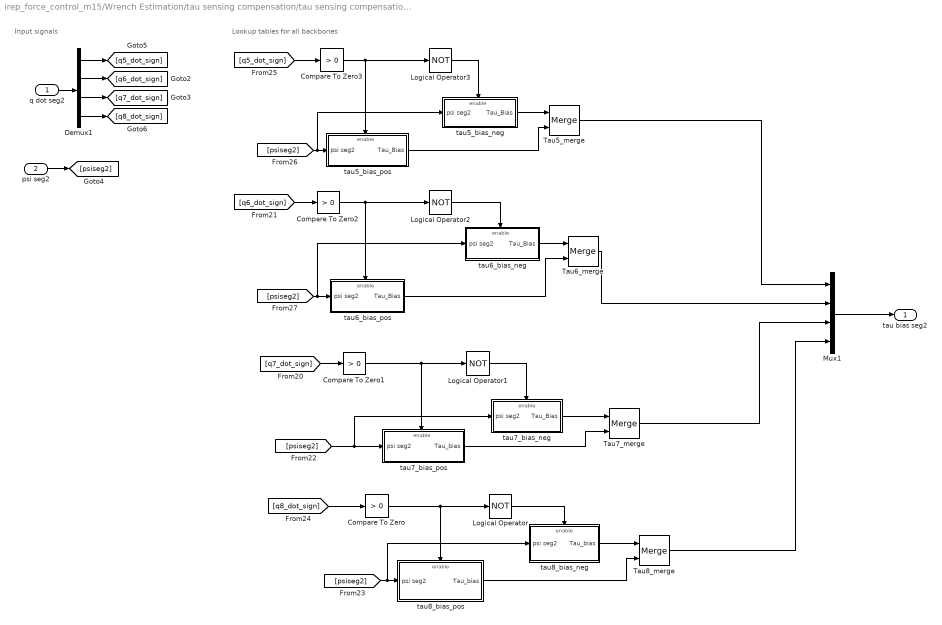
== system irep_force_control_m15/Wrench Estimation/tau sensing compensation/tau sensing compensation LUT/tau seg2 bias LUT ==
  note: Input signals
  note: Lookup tables for all backbones
  q dot seg2 : Inport
  psi seg2 : Inport  Port=2
  Compare To Zero{,1..3} (4 alike) : simulink/Logic and Bit Operations/Compare To Zero  relop=>  OutDataTypeStr=boolean
  Demux1 : Demux
  Logical Operator{,1..3} (4 alike) : Logic  Operator=NOT  AllPortsSameDT=off  OutDataTypeStr=boolean
  Mux1 : Mux
  Tau5_merge : Merge
  Tau6_merge : Merge
  Tau7_merge : Merge
  Tau8_merge : Merge
  tau5_bias_neg : Subsystem
  tau5_bias_pos : Subsystem
  tau6_bias_neg : Subsystem
  tau6_bias_pos : Subsystem
  tau7_bias_neg : Subsystem
  tau7_bias_pos : Subsystem
  tau8_bias_neg : Subsystem
  tau8_bias_pos : Subsystem
  tau bias seg2 : Outport
  wires:
  q dot seg2/1 -> Demux1/1
  Demux1/1 -> [q5_dot_sign]
  Demux1/2 -> [q6_dot_sign]
  Demux1/3 -> [q7_dot_sign]
  Demux1/4 -> [q8_dot_sign]
  psi seg2/1 -> [psiseg2]
  [q8_dot_sign] -> Compare To Zero/1
  Compare To Zero/1 -> Logical Operator/1, tau8_bias_pos/Enable
  Logical Operator/1 -> tau8_bias_neg/Enable
  tau8_bias_pos/1(Tau_bias) -> Tau8_merge/2
  tau8_bias_neg/1(Tau_bias) -> Tau8_merge/1
  Compare To Zero1/1 -> Logical Operator1/1, tau7_bias_pos/Enable
  Logical Operator1/1 -> tau7_bias_neg/Enable
  tau7_bias_pos/1(Tau_bias) -> Tau7_merge/2
  tau7_bias_neg/1(Tau_Bias) -> Tau7_merge/1
  [q7_dot_sign] -> Compare To Zero1/1
  [psiseg2] -> tau8_bias_neg/1(psi seg2), tau8_bias_pos/1(psi seg2)
  [psiseg2] -> tau7_bias_neg/1(psi seg2), tau7_bias_pos/1(psi seg2)
  [q6_dot_sign] -> Compare To Zero2/1
  Compare To Zero2/1 -> Logical Operator2/1, tau6_bias_pos/Enable
  Logical Operator2/1 -> tau6_bias_neg/Enable
  tau6_bias_pos/1(Tau_Bias) -> Tau6_merge/2
  tau6_bias_neg/1(Tau_Bias) -> Tau6_merge/1
  Compare To Zero3/1 -> Logical Operator3/1, tau5_bias_pos/Enable
  Logical Operator3/1 -> tau5_bias_neg/Enable
  tau5_bias_pos/1(Tau_Bias) -> Tau5_merge/2
  tau5_bias_neg/1(Tau_Bias) -> Tau5_merge/1
  [q5_dot_sign] -> Compare To Zero3/1
  Tau5_merge/1 -> Mux1/1
  Tau6_merge/1 -> Mux1/2
  Tau7_merge/1 -> Mux1/3
  Tau8_merge/1 -> Mux1/4
  Mux1/1 -> tau bias seg2/1
  [psiseg2] -> tau5_bias_neg/1(psi seg2), tau5_bias_pos/1(psi seg2)
  [psiseg2] -> tau6_bias_neg/1(psi seg2), tau6_bias_pos/1(psi seg2)

== system irep_force_control_m15/Trajectory Planner/Left Arm/High Level/Actuation Compensation/Compute Taus ==
  In1 : Inport
  In2 : Inport  Port=2
  Compute Tau : MATLAB Function  TreatAsAtomicUnit=on
  k_right : Constant  Value=k_right  SampleTime=dt
  tau : Outport
  wires:
  k_right/1 -> Compute Tau/3(k_right)
  In1/1 -> Compute Tau/1(GradU)
  Compute Tau/1(tau) -> tau/1
  In2/1 -> Compute Tau/2(conf_space)

== system irep_force_control_m15/Trajectory Planner/Left Arm/High Level/Actuation Compensation/Grad U1 ==
  conf space : Inport
  q : Inport  Port=2
  Compute grad U : MATLAB Function  TreatAsAtomicUnit=on
  Constant : Constant  Value=L1l  SampleTime=dt
  E_Y : Constant  Value=E_Y  SampleTime=dt
  Ip : Constant  Value=I1_primary+I2_primary  SampleTime=dt
  Is : Constant  Value=I1_secondary+I2_secondary  SampleTime=dt
  beta : Constant  Value=beta  SampleTime=dt
  r : Constant  Value=r  SampleTime=dt
  theta_0 : Constant  Value=theta0  SampleTime=dt
  grad_U : Outport
  wires:
  Constant/1 -> Compute grad U/3(L_p)
  beta/1 -> Compute grad U/9(beta)
  theta_0/1 -> Compute grad U/8(theta_0)
  r/1 -> Compute grad U/4(r)
  Ip/1 -> Compute grad U/6(Ip)
  E_Y/1 -> Compute grad U/5(E_Y)
  Compute grad U/1(grad_U) -> grad_U/1
  conf space/1 -> Compute grad U/1(conf_space)
  q/1 -> Compute grad U/2(q)
  Is/1 -> Compute grad U/7(Is)

== system irep_force_control_m15/Trajectory Planner/Left Arm/High Level/Actuation Compensation/Grad U2 ==
  conf space : Inport
  q : Inport  Port=2
  Compute grad U : MATLAB Function  TreatAsAtomicUnit=on
  Constant : Constant  Value=L2l  SampleTime=dt
  E_Y : Constant  Value=E_Y  SampleTime=dt
  Ip : Constant  Value=I2_primary  SampleTime=dt
  Is : Constant  Value=I2_secondary  SampleTime=dt
  beta : Constant  Value=beta  SampleTime=dt
  r : Constant  Value=r  SampleTime=dt
  theta_0 : Constant  Value=theta0  SampleTime=dt
  grad_U : Outport
  wires:
  Is/1 -> Compute grad U/7(Is)
  q/1 -> Compute grad U/2(q)
  conf space/1 -> Compute grad U/1(conf_space)
  Compute grad U/1(grad_U) -> grad_U/1
  E_Y/1 -> Compute grad U/5(E_Y)
  Ip/1 -> Compute grad U/6(Ip)
  r/1 -> Compute grad U/4(r)
  theta_0/1 -> Compute grad U/8(theta_0)
  beta/1 -> Compute grad U/9(beta)
  Constant/1 -> Compute grad U/3(L_p)

== system irep_force_control_m15/Trajectory Planner/Left Arm/High Level/Actuation Compensation/Parallelogram Backlash Compensatior ==
  q des : Inport
  Backlash Compensator : MATLAB Function  TreatAsAtomicUnit=on
  Bus Selector : BusSelector  OutputSignals=q2; q3
  Discrete Derivative : simulink/Discrete/Discrete Derivative  gainval=1.0  ICPrevScaledInput=0.0  InputProcessing=Inherited  OutMin=[]  OutMax=[]  OutDataType=fixdt(1, 16)  OutScaling=2^-10  DoSatur=off
  comp close : Constant  Value=0.5
  comp open : Constant  Value=-1
  epsilon : Outport
  wires:
  q des/1 -> Bus Selector/1
  Bus Selector/1 -> Discrete Derivative/1, Backlash Compensator/1(q_curr)  "<q2; q3>"
  Discrete Derivative/1 -> Backlash Compensator/2(q_dot_curr)  "q dot curr"
  Backlash Compensator/1(epsilon) -> epsilon/1
  comp open/1 -> Backlash Compensator/3(q2_comp_open)
  comp close/1 -> Backlash Compensator/4(q2_comp_close)

== system irep_force_control_m15/Trajectory Planner/Left Arm/High Level/Configuration Space/Parallelogram ==
  Enable : EnablePort
  5th Order Polynomial : Subsystem
  b_des : Constant  Value=[left_x0_parallelogram z0_parallelogram]  SampleTime=dt
  b1 : Outport
  wires:
  5th Order Polynomial/1(b) -> b1/1
  b_des/1 -> 5th Order Polynomial/1(b des)

== system irep_force_control_m15/Trajectory Planner/Left Arm/High Level/Configuration Space/Stem ==
  Enable : EnablePort
  5th Order Polynomial : Subsystem
  Terminator : Terminator
  enable : Constant  Value=0  SampleTime=dt
  psi des : Constant  Value=[pi/2;0;pi/2;0;0]  SampleTime=dt
  psi0 : Constant  Value=[pi/2;0;pi/2;0;0]  SampleTime=dt
  psi dot : Outport  InitialOutput=zeros(5,1)
  wires:
  enable/1 -> 5th Order Polynomial/3(enable)
  psi0/1 -> 5th Order Polynomial/2(psi0)
  psi des/1 -> 5th Order Polynomial/1(psi des)
  5th Order Polynomial/2(psi dot) -> psi dot/1
  5th Order Polynomial/1(psi) -> Terminator/1

== system irep_force_control_m15/Trajectory Planner/Left Arm/High Level/Inverse Istantaneous Kinematics/Coordination Module ==
  b1 : Inport
  q par : Inport  Port=2
  5-Bar Inverse Kinematics : MATLAB Function  TreatAsAtomicUnit=on
  Add : Sum  Inputs=+-  SampleTime=dt
  Coordination Block : MATLAB Function  TreatAsAtomicUnit=on
  L0 : Constant  Value=L_zeus  SampleTime=dt
  b0 : Constant  Value=[x0_parallelogram z0_parallelogram]  SampleTime=dt
  q1 : Outport
  "q2, q3" : Outport  Port=2
  wires:
  Add/1 -> "q2, q3"/1
  q par/1 -> Coordination Block/2(q_par)
  b1/1 -> Coordination Block/1(b1)
  Coordination Block/1(q1) -> q1/1
  5-Bar Inverse Kinematics/1(q) -> Add/2
  L0/1 -> Coordination Block/3(L0)
  b0/1 -> 5-Bar Inverse Kinematics/1(b1)
  Coordination Block/2(q23) -> Add/1

== system irep_force_control_m15/Trajectory Planner/Left Arm/High Level/Inverse Istantaneous Kinematics/Jaw Open//Close Module ==
  note: Temp fix,
      | teleop GP not working
  sensors : Inport
  Enable : EnablePort
  Bus Selector : BusSelector  OutputSignals=MSG_Type,gripper
  Jaw Open/Close : MATLAB Function  TreatAsAtomicUnit=on
  MTML_GP_max : Constant
  MTML_GP_min : Constant  Value=-1.3
  Unit Delay : UnitDelay  SampleTime=-1
  q9 : Outport
  wires:
  sensors/1 -> Bus Selector/1
  Jaw Open/Close/1(y) -> q9/1, Unit Delay/1
  MTML_GP_max/1 -> Jaw Open/Close/3(MTM_GP_max)
  MTML_GP_min/1 -> Jaw Open/Close/4(MTM_GP_min)
  Bus Selector/2 -> Jaw Open/Close/2(u)  "<gripper>"
  Bus Selector/1 -> Jaw Open/Close/1(MSG_valid)  "<MSG_Type>"
  Unit Delay/1 -> Jaw Open/Close/5(q9_prev)

== system irep_force_control_m15/Trajectory Planner/Left Arm/High Level/Task Space/Compute Weigths ==
  sensors : Inport
  conf space : Inport  Port=2
  Bus Selector : BusSelector  OutputSignals=b1 curr,psi curr
  Bus Selector1 : BusSelector  OutputSignals=foot switches
  joint limits : Constant  Value=[-x0_parallelogram_max -x0_parallelogram z0_parallelogram z0_parallelogram_max theta_min1 theta_max theta_min2 theta_max wrist_min wrist_max]  SampleTime=dt
  select weights : MATLAB Function  TreatAsAtomicUnit=on
  w min : Constant  Value=w_min  SampleTime=dt
  weights : Outport
  wires:
  joint limits/1 -> select weights/3(joint_limits)
  Bus Selector/1 -> select weights/1(b1)  "<b1 curr>"
  Bus Selector/2 -> select weights/2(psi)  "<psi curr>"
  conf space/1 -> Bus Selector/1
  select weights/1(W) -> weights/1
  w min/1 -> select weights/4(w_min)
  sensors/1 -> Bus Selector1/1
  Bus Selector1/1 -> select weights/5(foot_switches)  "<foot switches>"

== system irep_force_control_m15/Trajectory Planner/Left Arm/High Level/Task Space/Desired Twist Module ==
  note: Desired Twist Module v 1.1 - © 2011 Andrea Bajo, Nabil Simaan
  current pose : Inport
  des pose : Inport  Port=2
  Bus Selector1 : BusSelector  OutputSignals=p in world,R in world
  Bus Selector2 : BusSelector  OutputSignals=position,R,MSG_Type
  Compute Twist : MATLAB Function  TreatAsAtomicUnit=on
  Omega Max : Constant  Value=OmegaMax  SampleTime=dt
  Omega Min : Constant  Value=OmegaMin  SampleTime=dt
  Terminator : Terminator
  V Max : Constant  Value=Vmax  SampleTime=dt
  V Min : Constant  Value=Vmin  SampleTime=dt
  ang vel scale : Constant  Value=ang_vel_scale  SampleTime=dt
  lin vel scale : Constant  Value=lin_vel_scale  SampleTime=dt
  orientation epsilon : Constant  Value=orientation_epsilon  SampleTime=dt
  position epsilon : Constant  Value=position_epsilon  SampleTime=dt
  x des : Outport
  wires:
  Bus Selector1/1 -> Compute Twist/4(p_curr)  "<p in world>"
  Compute Twist/1(x_des) -> x des/1
  current pose/1 -> Bus Selector1/1
  Bus Selector1/2 -> Compute Twist/5(R_curr)  "<R in world>"
  Bus Selector2/1 -> Compute Twist/1(p_des)  "<position>"
  Bus Selector2/2 -> Compute Twist/2(R_des)  "<R>"
  des pose/1 -> Bus Selector2/1
  Bus Selector2/3 -> Compute Twist/3(MSG_Type)  "<MSG_Type>"
  V Max/1 -> Compute Twist/6(Vmax)
  Omega Max/1 -> Compute Twist/10(OmegaMax)
  V Min/1 -> Compute Twist/7(Vmin)
  Omega Min/1 -> Compute Twist/11(OmegaMin)
  position epsilon/1 -> Compute Twist/8(position_epsilon)
  orientation epsilon/1 -> Compute Twist/12(orientation_epsilon)
  lin vel scale/1 -> Compute Twist/9(lin_vel_scale)
  ang vel scale/1 -> Compute Twist/13(ang_vel_scale)
  Compute Twist/2(theta) -> Terminator/1

== system irep_force_control_m15/Trajectory Planner/Left Arm/High Level/Task Space/Direct Kinematics IREP ==
  "b1, psi" : Inport
  Bus Creator : BusCreator  Inputs=2
  Bus Selector : BusSelector  OutputSignals=Parker insertion stage,b1 curr,psi curr
  Direct Kinematic IREP : MATLAB Function  TreatAsAtomicUnit=on
  IREP parameters : Constant  Value=irep_parameters_left  SampleTime=dt
  Current Pose : Outport
  wires:
  "b1, psi"/1 -> Bus Selector/1
  Bus Selector/2 -> Direct Kinematic IREP/2(b1)  "<b1 curr>"
  Bus Selector/3 -> Direct Kinematic IREP/3(psi)  "<psi curr>"
  Direct Kinematic IREP/1(p) -> Bus Creator/1  "p in world"
  Direct Kinematic IREP/2(R) -> Bus Creator/2  "R in world"
  Bus Creator/1 -> Current Pose/1
  IREP parameters/1 -> Direct Kinematic IREP/4(parameters)
  Bus Selector/1 -> Direct Kinematic IREP/1(b0)  "<Parker insertion stage>"

== system irep_force_control_m15/Trajectory Planner/Left Arm/High Level/Task Space/Jxpsi Inverse IREP ==
  x des : Inport
  weights : Inport  Port=2
  "b1, psi" : Inport  Port=3
  Bus Selector1 : BusSelector  OutputSignals=Parker insertion stage,b1 curr,psi curr
  IREP parameters : Constant  Value=irep_parameters_left  SampleTime=dt
  Jxpsi Inverse IREP : MATLAB Function  TreatAsAtomicUnit=on
  epsilon : Constant  Value=epsilon_robust_inverse  SampleTime=dt
  max conf space speed : Constant  Value=max_conf_space_speed  SampleTime=dt
  conf dot des : Outport  PortDimensions=8
  wires:
  x des/1 -> Jxpsi Inverse IREP/1(x_des)
  Bus Selector1/3 -> Jxpsi Inverse IREP/4(psi)  "<psi curr>"
  Bus Selector1/2 -> Jxpsi Inverse IREP/3(b1)  "<b1 curr>"
  "b1, psi"/1 -> Bus Selector1/1
  Jxpsi Inverse IREP/1(conf_space_dot) -> conf dot des/1
  epsilon/1 -> Jxpsi Inverse IREP/7(epsilon_in)
  Bus Selector1/1 -> Jxpsi Inverse IREP/2(b0)  "<Parker insertion stage>"
  max conf space speed/1 -> Jxpsi Inverse IREP/8(max_ang_speed)
  weights/1 -> Jxpsi Inverse IREP/6(weights)
  IREP parameters/1 -> Jxpsi Inverse IREP/5(parameters)

== system irep_force_control_m15/Trajectory Planner/Left Arm/High Level/Task Space/Receive Desired Pose from MTM ==
  note: Telemanipulation Module v 1.0 - © COPYRIGHT 2010 Andrea Bajo, Nabil Simaan
  Master : Inport
  Bus Creator : BusCreator
  Bus Selector : BusSelector  OutputSignals=position,orientation (quat),MSG_Type,gripper
  Quaternion To Rotation : MATLAB Function  TreatAsAtomicUnit=on
  "pose, flags" : Outport
  wires:
  Bus Creator/1 -> "pose, flags"/1
  Master/1 -> Bus Selector/1
  Bus Selector/1 -> Bus Creator/1  "<position>"
  Quaternion To Rotation/1(R) -> Bus Creator/2
  Bus Selector/2 -> Quaternion To Rotation/1(quat)  "<orientation (quat)>"
  Bus Selector/3 -> Bus Creator/3  "<MSG_Type>"
  Bus Selector/4 -> Bus Creator/4  "<gripper>"

== system irep_force_control_m15/Trajectory Planner/Left Arm/High Level/Task Space/right task space scope ==
  In : Inport
  Bus Selector7 : BusSelector  OutputSignals=position,R,gripper,MSG_Type
  Gain : Gain
  Mux : Mux  Inputs=5
  R_to_axis_angle1 : MATLAB Function  TreatAsAtomicUnit=on
  left task space : slrtlib/Displays and Logging/Scope   scopeno=18  scopetype=Host  autostart=on  viewmode=Numerical  formatstr=scope_format_left_task_space_des  grid=on  ylimits=[0,0]  nosamples=10  noprepostsamples=0  interleave=1  triggermode=FreeRun  triggersignal=1  trigsignalfromport=off  triggerlevel=0.0  triggerslope=Either  triggerscope=1  triggersample=0  filename=weights1.dat  mode=Lazy  writesize=512  autorestart=off  dynamicfilemode=off  maxwritefilesize=512*1024^2
  wires:
  Mux/1 -> Gain/1
  In/1 -> Bus Selector7/1
  Bus Selector7/2 -> R_to_axis_angle1/1(R)  "<R>"
  Gain/1 -> left task space/1
  Bus Selector7/1 -> Mux/1  "<position>"
  R_to_axis_angle1/1(n_vec) -> Mux/2
  R_to_axis_angle1/2(theta) -> Mux/3
  Bus Selector7/3 -> Mux/4  "<gripper>"
  Bus Selector7/4 -> Mux/5  "<MSG_Type>"

== system irep_force_control_m15/Trajectory Planner/Left Arm/Low Level/Home Procedure/Fine Homing - Integral Control ==
  error : Inport
  Enable : EnablePort  StatesWhenEnabling=reset
  Discrete-Time Integrator : DiscreteIntegrator  SampleTime=dt  LimitOutput=on  UpperSaturationLimit=8  LowerSaturationLimit=-8
  Integral Gain : Gain  Gain=diag(LeftArmHomingIntGain)  Multiplication=Matrix(K*u)  SampleTime=dt
  q_des_fine : Outport  InitialOutput=zeros(9,1)
  wires:
  error/1 -> Integral Gain/1
  Discrete-Time Integrator/1 -> q_des_fine/1
  Integral Gain/1 -> Discrete-Time Integrator/1

== system irep_force_control_m15/Trajectory Planner/Left Arm/Low Level/Home Procedure/Homing Flags ==
  u : Inport
  Homing Completion : MATLAB Function  TreatAsAtomicUnit=on
  HomingFineEps : Constant  Value=HomingFineEps  SampleTime=dt
  Terminator1 : Terminator
  Unit Delay : UnitDelay  InitialCondition=zeros(9,1)  SampleTime=-1
  dt : Constant  Value=dt  SampleTime=dt
  wires:
  Homing Completion/1(Homed) -> Terminator1/1
  HomingFineEps/1 -> Homing Completion/2(EPS)
  u/1 -> Homing Completion/1(u)
  Homing Completion/2(Homed_T) -> Unit Delay/1
  Unit Delay/1 -> Homing Completion/4(Homed_T_prev)
  dt/1 -> Homing Completion/3(dt)

== system irep_force_control_m15/Trajectory Planner/Right Arm/High Level/Actuation Compensation/Compute Taus ==
  In1 : Inport
  In2 : Inport  Port=2
  Compute Tau : MATLAB Function  TreatAsAtomicUnit=on
  k_right : Constant  Value=k_right  SampleTime=dt
  tau : Outport
  wires:
  k_right/1 -> Compute Tau/3(k_right)
  In1/1 -> Compute Tau/1(GradU)
  Compute Tau/1(tau) -> tau/1
  In2/1 -> Compute Tau/2(conf_space)

== system irep_force_control_m15/Trajectory Planner/Right Arm/High Level/Actuation Compensation/Grad U1 ==
  conf space : Inport
  q : Inport  Port=2
  Compute grad U : MATLAB Function  TreatAsAtomicUnit=on
  Constant : Constant  Value=L1r  SampleTime=dt
  E_Y : Constant  Value=E_Y  SampleTime=dt
  Ip : Constant  Value=I1_primary+I2_primary  SampleTime=dt
  Is : Constant  Value=I1_secondary+I2_secondary  SampleTime=dt
  beta : Constant  Value=beta  SampleTime=dt
  r : Constant  Value=r  SampleTime=dt
  theta_0 : Constant  Value=theta0  SampleTime=dt
  grad_U : Outport
  wires:
  Constant/1 -> Compute grad U/3(L_p)
  beta/1 -> Compute grad U/9(beta)
  theta_0/1 -> Compute grad U/8(theta_0)
  r/1 -> Compute grad U/4(r)
  Ip/1 -> Compute grad U/6(Ip)
  E_Y/1 -> Compute grad U/5(E_Y)
  Compute grad U/1(grad_U) -> grad_U/1
  conf space/1 -> Compute grad U/1(conf_space)
  q/1 -> Compute grad U/2(q)
  Is/1 -> Compute grad U/7(Is)
